simulink model "my_model"  (R2020b)
settings: Solver=ode8  StartTime=0.0  StopTime=3  FixedStep=0.005  RelTol=1e-3
values from neighbouring files (symbols this model uses):
  g1 = [-1 0 1]    [Model_3D_file.m]
  g2 = [-1 0.6 1]    [Model_3D_file.m]
  left_0 = [0 0 0]    [Model_3D_file.m]
  right_0 = [0 0.6 0]    [Model_3D_file.m]
  tau1 = 3    [Model_3D_file.m]
  x1_0 = [0 0.2 0]    [Model_3D_file.m]
  x2_0 = [0 0.4 0]    [Model_3D_file.m]
undefined symbols (not defined in the file or in its folder): Am, b1, b2, b3, Bm, cc, D, gamma1, gamma2, K, k1, k2, k3, m1, m2, weight, width
settings Model: Creator=nathan  LastModifiedBy=10788
settings OptimizationCC: DefaultParameterBehavior=Inlined  EnhancedBackFolding=on  PassReuseOutputArgsAs=Individual arguments  ZeroExternalMemoryAtStartup=off  ZeroInternalMemoryAtStartup=off  OptimizeBlockOrder=speed  DifferentSizesBufferReuse=on  OptimizationCustomize=off  EfficientTunableParamExpr=on
settings DebuggingCC: ParameterTunabilityLossMsg=error
settings SFSimCC: MATLABDynamicMemAlloc=off  SimTargetLang=C++
settings RTWCC: Description=Create Visual C/C++ Solution File for Embedded Coder  SystemTargetFile=ert.tlc  GenCodeOnly=on  TemplateMakefile=RTW.MSVCBuild  GenerateReport=on  IncludeHyperlinkInReport=on  LaunchReport=on  TargetLang=C++  GenerateTraceInfo=on  GenerateTraceReport=on  GenerateTraceReportSl=on  GenerateTraceReportSf=on  GenerateTraceReportEml=on
settings CodeAppCC: ForceParamTrailComments=on  IgnoreCustomStorageClasses=off  OperatorAnnotations=on  SimulinkDataObjDesc=on  SFDataObjDesc=on  InsertBlockDesc=on
settings ERTTargetCC: TargetLangStandard=C++03 (ISO)  GenerateSampleERTMain=on  CodeInterfacePackaging=C++ class  SupportContinuousTime=on  InlinedParameterPlacement=NonHierarchical  RootIOFormat=Structure reference  ERTCustomFileTemplate=example_file_process.tlc

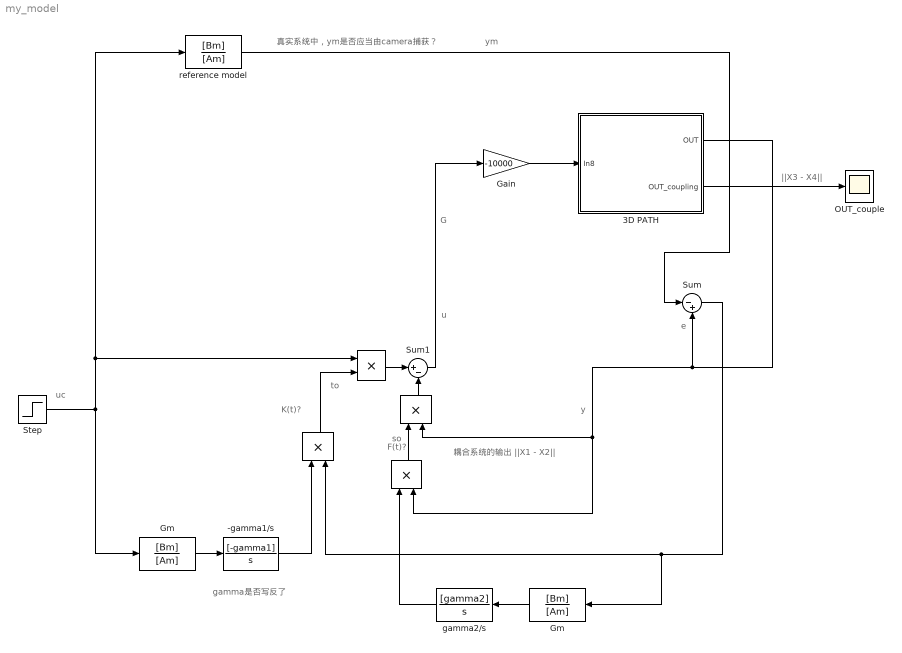
== system my_model ==
  note: gamma是否写反了
  note: F(t)?
  note: K(t)?
  note: 真实系统中，ym是否应当由camera捕获？
  note: 耦合系统的输出 ||X1 - X2||
  note: ||X3 - X4||
  note: y
  note: u
  note: e
  note: so
  note: to
  note: uc
  note: ym
  note: G
  " " : Product
  " " : Product
  "  " : Product
  "     " : Product
  -gamma1/s : TransferFcn  Numerator=[-gamma1]  Denominator=[1 0]
  3D PATH : Subsystem
  Gain : Gain  Gain=-10000
  "Gm " : TransferFcn  Numerator=[Bm]  Denominator=[Am]
  "Gm  " : TransferFcn  Numerator=[Bm]  Denominator=[Am]
  OUT_couple : Scope
  Step : Step  Time=0  After=0.2  SampleTime=0
  Sum : Sum  Inputs=|-+
  Sum1 : Sum  Inputs=|+-
  gamma2/s : TransferFcn  Numerator=[gamma2]  Denominator=[1 0]
  reference model : TransferFcn  Numerator=[Bm]  Denominator=[Am]
  wires:
  3D PATH/1(OUT) -> "  "/2, " "/2, Sum/2
  " "/1 -> Sum1/2
  Step/1 -> "Gm  "/1, reference model/1, "     "/1
  "  "/1 -> " "/1
  Gain/1 -> 3D PATH/1(In8)
  Sum1/1 -> Gain/1
  -gamma1/s/1 -> " "/1
  " "/1 -> "     "/2
  "Gm "/1 -> gamma2/s/1
  "     "/1 -> Sum1/1
  reference model/1 -> Sum/1
  gamma2/s/1 -> "  "/1
  Sum/1 -> "Gm "/1, " "/2
  "Gm  "/1 -> -gamma1/s/1
  3D PATH/2(OUT_coupling) -> OUT_couple/1

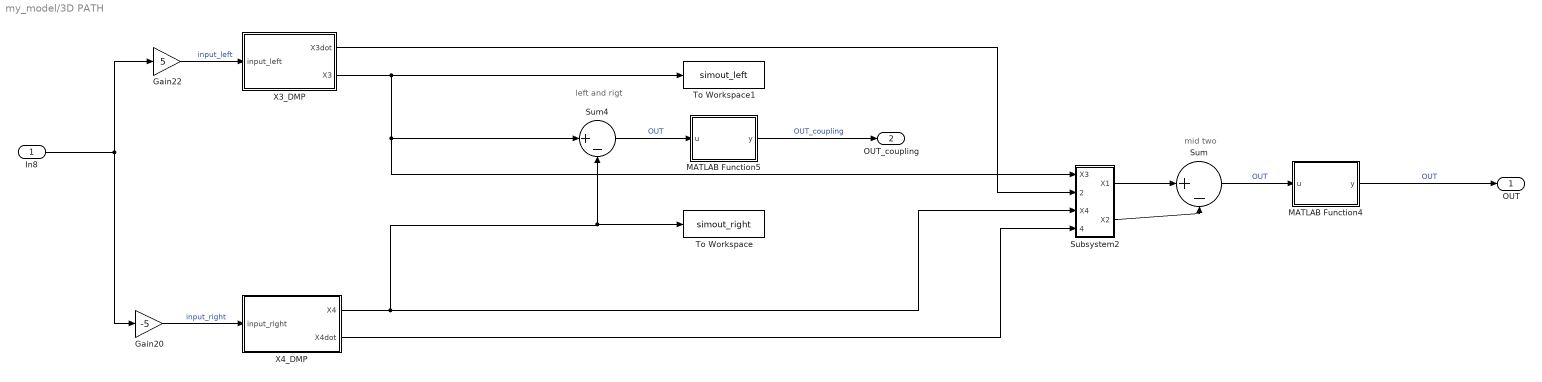
== system my_model/3D PATH ==
  note: mid two
  note: left and rigt
  In8 : Inport
  Gain20 : Gain  Gain=-5
  Gain22 : Gain  Gain=5
  MATLAB Function4 : MATLAB Function  TreatAsAtomicUnit=on
  MATLAB Function5 : MATLAB Function  TreatAsAtomicUnit=on
  Subsystem2 : Subsystem
  Sum : Sum  Inputs=|+-
  Sum4 : Sum  Inputs=|+-
  To Workspace : ToWorkspace  VariableName=simout_right  SaveFormat=Timeseries  SampleTime=-1
  To Workspace1 : ToWorkspace  VariableName=simout_left  SaveFormat=Timeseries  SampleTime=-1
  X3_DMP : Subsystem
  X4_DMP : Subsystem
  OUT : Outport
  OUT_coupling : Outport  Port=2
  wires:
  MATLAB Function5/1(y) -> OUT_coupling/1  "OUT_coupling"
  In8/1 -> Gain20/1, Gain22/1
  Sum4/1 -> MATLAB Function5/1(u)  "OUT"
  Sum/1 -> MATLAB Function4/1(u)  "OUT"
  MATLAB Function4/1(y) -> OUT/1  "OUT"
  X3_DMP/2(X3) -> Subsystem2/1(X3), Sum4/1, To Workspace1/1
  Gain22/1 -> X3_DMP/1(input_left)  "input_left"
  X4_DMP/1(X4) -> Subsystem2/3(X4), Sum4/2, To Workspace/1
  Gain20/1 -> X4_DMP/1(input_right)  "input_right"
  X3_DMP/1(X3dot) -> Subsystem2/2(X3dot)
  X4_DMP/2(X4dot) -> Subsystem2/4(X4dot)
  Subsystem2/1(X1) -> Sum/1
  Subsystem2/2(X2) -> Sum/2

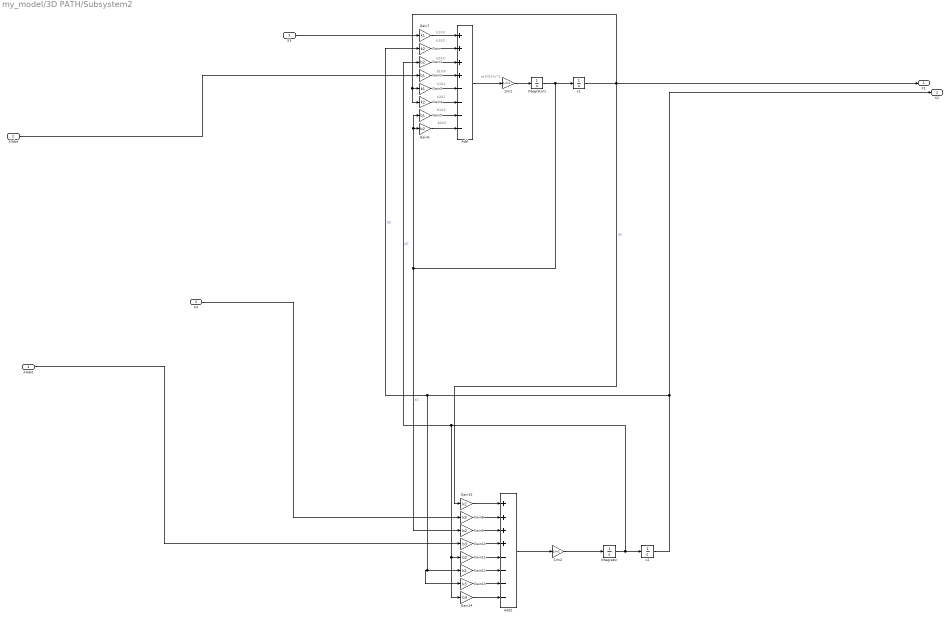
== system my_model/3D PATH/Subsystem2 ==
  note: m1*X1*s^2
  note: k1X3
  note: k2X2
  note: b2X2'
  note: b1X3'
  note: k1X1
  note: k2X1
  note: b1X1'
  note: b2X1'
  X3 : Inport
  X3dot : Inport  Port=2
  X4 : Inport  Port=3
  X4dot : Inport  Port=4
  1/m1 : Gain  Gain=1/m1
  1/m2 : Gain  Gain=1/m2
  Add : Sum  Inputs=++++----
  Add1 : Sum  Inputs=++++----
  Gain{,4,12,15} (4 alike) : Gain  Gain=k2
  Gain{1,6,9,11} (4 alike) : Gain  Gain=b2
  Gain10 : Gain  Gain=b3
  Gain13 : Gain  Gain=k3
  Gain14 : Gain  Gain=b3
  Gain2 : Gain  Gain=b1
  Gain3 : Gain  Gain=k1
  Gain5 : Gain  Gain=b1
  Gain7 : Gain  Gain=k1
  Gain8 : Gain  Gain=k3
  Integrator : Integrator
  Integrator1 : Integrator
  x1 : Integrator  InitialCondition=x1_0
  x2 : Integrator  InitialCondition=x2_0
  X1 : Outport
  X2 : Outport  Port=2
  wires:
  Integrator1/1 -> x1/1, Gain9/1, Gain5/1, Gain6/1  "x1'"
  Gain8/1 -> Add1/2
  x2/1 -> X2/1, Gain13/1, Gain12/1, Gain/1  "X2"
  x1/1 -> X1/1, Gain15/1, Gain4/1, Gain3/1  "X1"
  Gain14/1 -> Add1/8
  1/m1/1 -> Integrator1/1
  Gain3/1 -> Add/5
  Integrator/1 -> x2/1, Gain1/1, Gain14/1, Gain11/1  "x2'"
  Gain/1 -> Add/2
  Gain5/1 -> Add/7
  1/m2/1 -> Integrator/1
  Gain7/1 -> Add/1
  Add/1 -> 1/m1/1
  Gain15/1 -> Add1/1
  Gain2/1 -> Add/4
  Gain1/1 -> Add/3
  Gain6/1 -> Add/8
  Gain4/1 -> Add/6
  Gain9/1 -> Add1/3
  X3/1 -> Gain7/1
  Gain11/1 -> Add1/5
  Gain13/1 -> Add1/7
  Gain12/1 -> Add1/6
  Gain10/1 -> Add1/4
  X4/1 -> Gain8/1
  Add1/1 -> 1/m2/1
  X4dot/1 -> Gain10/1
  X3dot/1 -> Gain2/1

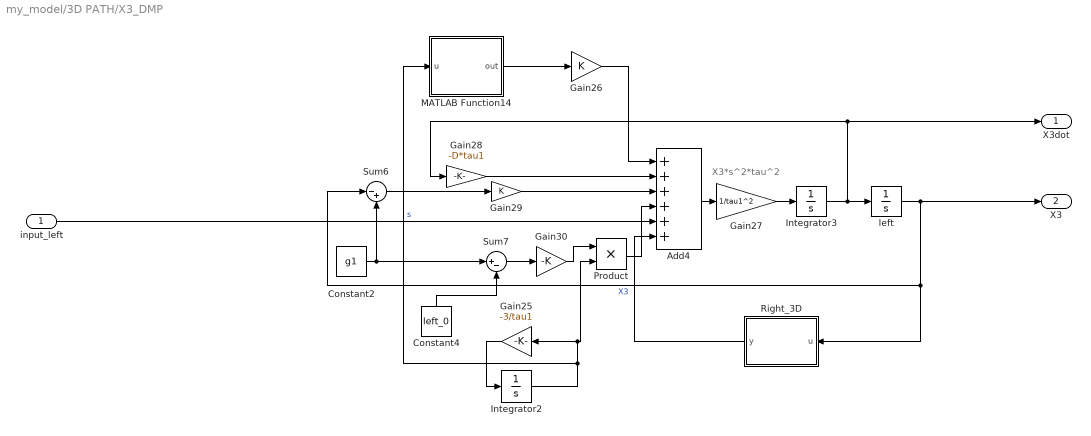
== system my_model/3D PATH/X3_DMP ==
  note: X3*s^2*tau^2
  input_left : Inport
  Add4 : Sum  Inputs=++++++
  Constant2 : Constant  Value=g1
  Constant4 : Constant  Value=left_0
  Gain25 : Gain  Gain=-3/tau1
  Gain26 : Gain  Gain=K
  Gain27 : Gain  Gain=1/tau1^2
  Gain28 : Gain  Gain=-D*tau1
  Gain29 : Gain  Gain=K
  Gain30 : Gain  Gain=-K
  Integrator2 : Integrator  InitialCondition=1
  Integrator3 : Integrator
  MATLAB Function14 : MATLAB Function  TreatAsAtomicUnit=on
  Product : Product
  Right_3D : MATLAB Function  TreatAsAtomicUnit=on
  Sum6 : Sum  Inputs=|-+
  Sum7 : Sum  Inputs=|+-
  left : Integrator  InitialCondition=left_0
  X3dot : Outport
  X3 : Outport  Port=2
  wires:
  Constant2/1 -> Sum7/1, Sum6/2
  Gain25/1 -> Integrator2/1
  Gain30/1 -> Product/1
  Sum6/1 -> Gain29/1
  Constant4/1 -> Sum7/2
  MATLAB Function14/1(out) -> Gain26/1
  Right_3D/1(y) -> Add4/6
  input_left/1 -> Add4/5
  Add4/1 -> Gain27/1
  Integrator2/1 -> MATLAB Function14/1(u), Product/2, Gain25/1  "s"
  Gain28/1 -> Add4/2
  left/1 -> Right_3D/1(u), Sum6/1, X3/1  "X3"
  Sum7/1 -> Gain30/1
  Gain29/1 -> Add4/3
  Gain27/1 -> Integrator3/1
  Integrator3/1 -> Gain28/1, X3dot/1, left/1
  Product/1 -> Add4/4
  Gain26/1 -> Add4/1

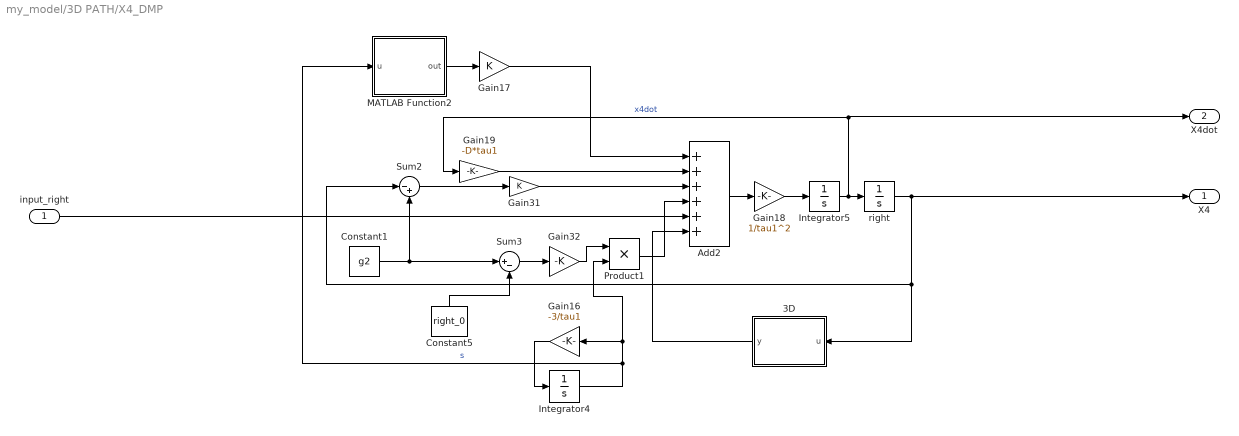
== system my_model/3D PATH/X4_DMP ==
  input_right : Inport
  3D : MATLAB Function  TreatAsAtomicUnit=on
  Add2 : Sum  Inputs=++++++
  Constant1 : Constant  Value=g2
  Constant5 : Constant  Value=right_0
  Gain16 : Gain  Gain=-3/tau1
  Gain17 : Gain  Gain=K
  Gain18 : Gain  Gain=1/tau1^2
  Gain19 : Gain  Gain=-D*tau1
  Gain31 : Gain  Gain=K
  Gain32 : Gain  Gain=-K
  Integrator4 : Integrator  InitialCondition=1
  Integrator5 : Integrator
  MATLAB Function2 : MATLAB Function  TreatAsAtomicUnit=on
  Product1 : Product
  Sum2 : Sum  Inputs=|-+
  Sum3 : Sum  Inputs=|+-
  right : Integrator  InitialCondition=right_0
  X4 : Outport
  X4dot : Outport  Port=2
  wires:
  Integrator5/1 -> X4dot/1, Gain19/1, right/1  "x4dot"
  Sum2/1 -> Gain31/1
  Gain32/1 -> Product1/1
  Gain17/1 -> Add2/1
  3D/1(y) -> Add2/6
  Sum3/1 -> Gain32/1
  Gain19/1 -> Add2/2
  MATLAB Function2/1(out) -> Gain17/1
  Gain16/1 -> Integrator4/1
  right/1 -> 3D/1(u), Sum2/1, X4/1
  Integrator4/1 -> Product1/2, Gain16/1, MATLAB Function2/1(u)  "s"
  Constant1/1 -> Sum3/1, Sum2/2
  Constant5/1 -> Sum3/2
  Gain18/1 -> Integrator5/1
  Product1/1 -> Add2/4
  Gain31/1 -> Add2/3
  Add2/1 -> Gain18/1
  input_right/1 -> Add2/5

== matlab function my_model/3D PATH/X4_DMP/3D ==
  data: u input; y output
function y = fcn(u)

n_dim=3;
n_obt=2;
phi=zeros(n_dim,1);     % 3行1列
phi_tal=zeros(n_dim,1); % 2行1列

% 障碍物1
x_c_1 = 0.2;
y_c_1 = 0.8;
z_c_1 = 0.4;
a_1 = .1;
b_1 = .2;
c_1 = .1;

% 障碍物2
x_c_2 = -0.4;
y_c_2 = 1.2;
z_c_2 = 0.8;
a_2 = 0.15;
b_2 = 0.15;
c_2 = .2;

center=[x_c_1 y_c_1 z_c_1;
    x_c_2 y_c_2 z_c_2
];
axis=[a_1 b_1 c_1;
    a_2 b_2 c_2
];

% center=center(:,[2 1]);
% axis=axis(:,[2 1]);

%%%%%%%%%%%%%

for j=1:n_obt % 障碍物数量
    K = 0;
    for i = 1:n_dim % 坐标维度
        K =K+( (u(i) - center(j,i)) / axis(j,i)) ^2;
    end
    K = K - 1;

    for i = 1:n_dim
        phi(i) = (u(i) - center(j,i)) / axis(j,i) ^2;
    end

    phi = phi * ( exp(-K)) * (1 / K + 1 / K / K) * 2;
    phi_tal=phi_tal+phi;
end

y = phi_tal;

== matlab function my_model/3D PATH/X3_DMP/MATLAB Function14 ==
  data: u input; out output; width parameter; weight parameter; cc parameter
function out = fcn(u, width, weight, cc)


% if(u>2.5)
%     y=1;
% elseif(u>=0&&u<=2.5)
%     y=0;
% else
%         y=-1;
% end


tem=exp(-width.*(u-cc).^2)';
y=(weight*tem*u)/sum(tem) ;

out = y;

== matlab function my_model/3D PATH/X4_DMP/MATLAB Function2 ==
  data: u input; out output; width parameter; weight parameter; cc parameter
function out = fcn(u, width, weight, cc)


% if(u>2.5)
%     y=1;
% elseif(u>=0&&u<=2.5)
%     y=0;
% else
%         y=-1;
% end


tem=exp(-width.*(u-cc).^2)';
y=(weight*tem*u)/sum(tem) ;

out = y;

== matlab function my_model/3D PATH/MATLAB Function4 ==
  data: u input; y output
function y = fcn(u)

y = norm(u);

== matlab function my_model/3D PATH/MATLAB Function5 ==
  data: u input; y output
function y = fcn(u)

y = norm(u);

== matlab function my_model/3D PATH/X3_DMP/Right_3D ==
  data: u input; y output
function y = fcn(u)

n_dim=3;
n_obt=1;
phi=zeros(n_dim,1);
phi_tal=zeros(n_dim,1);

x_c_1 = 0.15;
y_c_1 = 0.2;
z_c_1 = 0.4;
a_1 = .1;
b_1 = .1;
c_1 = .1;

x_c_2 = -0.4;
y_c_2 = 1.1;
z_c_2 = 0.8;
a_2 = 0.15;
b_2 = 0.15;
c_2 = .2;

% center=[x_c_1 y_c_1;
%     x_c_2 y_c_2];
% axis=[a_1 b_1;
%     a_2 b_2];

center=[x_c_1 y_c_1 z_c_1;
    x_c_2 y_c_2 z_c_2
];
axis=[a_1 b_1 c_1;
    a_2 b_2 c_2
];

% center=center(:,[2 1]);
% axis=axis(:,[2 1]);

%%%%%%%%%%%%%

for j=1:n_obt
    
    
    K = 0;
for i = 1:n_dim
    
    K =K+( (u(i) - center(j,i)) / axis(j,i)) ^2;
    
end
K = K - 1;

for i = 1:n_dim
    phi(i) = (u(i) - center(j,i)) / axis(j,i) ^2;
   
end

phi =phi * ( exp(-K)) * (1 / K + 1 / K / K) * 2;
      
phi_tal=phi_tal+phi;
end


y = phi_tal;
